simulink model "NREL_Turbine"  (R2020a)
settings: Solver=VariableStepAuto  StartTime=0.0  StopTime=100  RelTol=1e-3
undefined symbols (not defined in the file): Pb, w_HS
libraries: libturbines x1
settings Model: Creator=dvapo  LastModifiedBy=joakbj

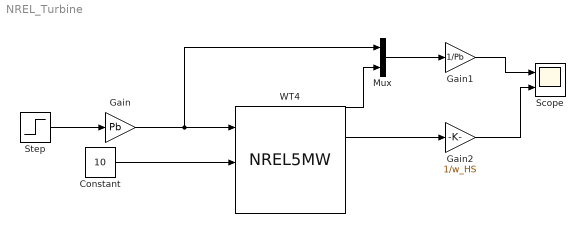
== system NREL_Turbine ==
  Constant : Constant  Value=10
  Gain : Gain  Gain=Pb
  Gain1 : Gain  Gain=1/Pb
  Gain2 : Gain  Gain=1/w_HS
  Mux : Mux  Inputs=2
  Scope : Scope  NumInputPorts=2
  Step : Step  SampleTime=0
  WT4 : libturbines/NREL5MW  w_gen_ini=50  beta_ini=0  auto=off  torq_ini=0
  wires:
  Step/1 -> Gain/1
  Gain/1 -> Mux/1, WT4/1
  Constant/1 -> WT4/2
  WT4/1 -> Mux/2
  Mux/1 -> Gain1/1
  WT4/3 -> Gain2/1
  Gain1/1 -> Scope/1
  Gain2/1 -> Scope/2
